simulink model "sampleModel7293_pp_1_1"  (R2018a)
settings: Solver=VariableStepAuto  StartTime=0.0  StopTime=10.0  RelTol=1e-3
undefined symbols (not defined in the file): DiscIntNeverNeededParam
libraries: simulink x367
(part 12 of 12)

== system sampleModel7293_pp_1_1/cfblk187/cfblk12/cfblk3 ==
  emi_1187 : Inport
  emi_1188 : Inport  Port=2
  Action Port : ActionPort  ActionType=then
  cfblk3 : simulink/Continuous/PID Controller (2DOF)  Controller=PID  TimeDomain=Discrete-time  SampleTime=-1  IntegratorMethod=Forward Euler  FilterMethod=Forward Euler  Form=Parallel  UseFilter=on  ControllerParametersSource=internal  P=1  I=1  D=0  N=100  b=1  c=1  InitialConditionSource=internal  InitialConditionForIntegrator=0  InitialConditionForFilter=0  ExternalReset=none  LimitOutput=off  UpperSaturationLimit=inf  LowerSaturationLimit=-inf  LinearizeAsGain=off  AntiWindupMode=none  Kb=1  TrackingMode=off  Kt=1  PParamMin=[]  PParamMax=[]  IParamMin=[]  IParamMax=[]  DParamMin=[]  DParamMax=[]  NParamMin=[]  NParamMax=[]  bParamMin=[]  bParamMax=[]  cParamMin=[]  cParamMax=[]  KbParamMin=[]  KbParamMax=[]  KtParamMin=[]  KtParamMax=[]  POutMin=[]  POutMax=[]  IOutMin=[]  IOutMax=[]  DOutMin=[]  DOutMax=[]  NOutMin=[]  NOutMax=[]  bOutMin=[]  bOutMax=[]  cOutMin=[]  cOutMax=[]  KbOutMin=[]  KbOutMax=[]  KtOutMin=[]  KtOutMax=[]  IntegratorOutMin=[]  IntegratorOutMax=[]  FilterOutMin=[]  FilterOutMax=[]  SumOutMin=[]  SumOutMax=[]  Sum1OutMin=[]  Sum1OutMax=[]  Sum2OutMin=[]  Sum2OutMax=[]  Sum3OutMin=[]  Sum3OutMax=[]  SumI1OutMin=[]  SumI1OutMax=[]  SumI2OutMin=[]  SumI2OutMax=[]  SumI3OutMin=[]  SumI3OutMax=[]  SumDOutMin=[]  SumDOutMax=[]  SaturationOutMin=[]  SaturationOutMax=[]  IntegratorContinuousStateAttributes=''  IntegratorStateMustResolveToSignalObject=off  IntegratorRTWStateStorageClass=Auto  FilterContinuousStateAttributes=''  FilterStateMustResolveToSignalObject=off  FilterRTWStateStorageClass=Auto  DifferentiatorICPrevScaledInput=0  DifferentiatorOutMin=[]  DifferentiatorOutMax=[]  FilterDiffOutCoefMin=[]  FilterDiffOutCoefMax=[]  SumDenOutMin=[]  SumDenOutMax=[]  SumNumOutMin=[]  SumNumOutMax=[]  ReciprocalOutMin=[]  ReciprocalOutMax=[]  DivideOutMin=[]  DivideOutMax=[]  TunerSelectOption=Transfer Function Based (PID Tuner App)
  emi_1189 : Outport
  wires:
  emi_1187/1 -> cfblk3/1
  emi_1188/1 -> cfblk3/2
  cfblk3/1 -> emi_1189/1

== system sampleModel7293_pp_1_1/cfblk187/cfblk12/cfblk7 ==
  emi_322 : Inport
  Action Port : ActionPort  ActionType=then
  cfblk7 : DiscreteTransferFcn
  emi_323 : Outport
  wires:
  emi_322/1 -> cfblk7/1
  cfblk7/1 -> emi_323/1

== system sampleModel7293_pp_1_1/cfblk187/cfblk12/emi_1190 ==
  Action Port : ActionPort  ActionType=else
  emi_1191 : Assertion

== system sampleModel7293_pp_1_1/cfblk187/cfblk12/emi_324 ==
  Action Port : ActionPort  ActionType=else
  emi_325 : Assertion

== system sampleModel7293_pp_1_1/cfblk189/cfblk16/cfblk8 ==
  emi_903 : Inport
  Action Port : ActionPort  ActionType=then
  cfblk8 : simulink/Discrete/Transfer Fcn First Order  PoleZ=0.95  ICPrevOutput=0.0  DoSatur=off
      settings: SourceProductName=Simulink
  emi_904 : Outport
  wires:
  emi_903/1 -> cfblk8/1
  cfblk8/1 -> emi_904/1

== system sampleModel7293_pp_1_1/cfblk189/cfblk16/emi_905 ==
  Action Port : ActionPort  ActionType=else
  emi_906 : Assertion

== system sampleModel7293_pp_1_1/cfblk189/cfblk17/cfblk13 ==
  emi_359 : Inport
  Action Port : ActionPort  ActionType=then
  cfblk13 : simulink/Discrete/Difference  ICPrevInput=0.0  OutMin=[]  OutMax=[]  OutDataTypeStr=double  OutputDataTypeScalingMode=double  OutDataType=fixdt(1, 16)  OutScaling=2^-10  DoSatur=off
  emi_360 : Outport
  wires:
  emi_359/1 -> cfblk13/1
  cfblk13/1 -> emi_360/1

== system sampleModel7293_pp_1_1/cfblk189/cfblk17/cfblk4 ==
  emi_810 : Inport
  Action Port : ActionPort  ActionType=then
  cfblk4 : DiscreteStateSpace  SampleTime=-1
  emi_811 : Outport
  wires:
  emi_810/1 -> cfblk4/1
  cfblk4/1 -> emi_811/1

== system sampleModel7293_pp_1_1/cfblk189/cfblk17/cfblk9 ==
  emi_366 : Inport
  Action Port : ActionPort  ActionType=then
  cfblk9 : DiscreteTransferFcn
  emi_367 : Outport
  wires:
  emi_366/1 -> cfblk9/1
  cfblk9/1 -> emi_367/1

== system sampleModel7293_pp_1_1/cfblk189/cfblk17/emi_361 ==
  Action Port : ActionPort  ActionType=else
  emi_362 : Assertion

== system sampleModel7293_pp_1_1/cfblk189/cfblk17/emi_368 ==
  Action Port : ActionPort  ActionType=else
  emi_369 : Assertion

== system sampleModel7293_pp_1_1/cfblk189/cfblk17/emi_812 ==
  Action Port : ActionPort  ActionType=else
  emi_813 : Assertion

== system sampleModel7293_pp_1_1/cfblk190/cfblk10/cfblk10 ==
  emi_523 : Inport
  emi_524 : Inport  Port=2
  Action Port : ActionPort  ActionType=then
  cfblk10 : Delay  DelayLengthSource=Input port
      settings: InputPortMap=u0,p1
  emi_525 : Outport
  wires:
  emi_523/1 -> cfblk10/1
  emi_524/1 -> cfblk10/2
  cfblk10/1 -> emi_525/1

== system sampleModel7293_pp_1_1/cfblk190/cfblk10/cfblk16 ==
  emi_545 : Inport
  Action Port : ActionPort  ActionType=then
  cfblk16 : Delay
  emi_546 : Outport
  wires:
  emi_545/1 -> cfblk16/1
  cfblk16/1 -> emi_546/1

== system sampleModel7293_pp_1_1/cfblk190/cfblk10/cfblk4 ==
  emi_952 : Inport
  Action Port : ActionPort  ActionType=then
  cfblk4 : DiscreteFir
  emi_953 : Outport
  wires:
  emi_952/1 -> cfblk4/1
  cfblk4/1 -> emi_953/1

== system sampleModel7293_pp_1_1/cfblk190/cfblk10/cfblk5 ==
  emi_1223 : Inport
  Action Port : ActionPort  ActionType=then
  cfblk5 : simulink/Continuous/PID Controller  Controller=PID  TimeDomain=Discrete-time  SampleTime=-1  IntegratorMethod=Forward Euler  FilterMethod=Forward Euler  Form=Parallel  UseFilter=on  ControllerParametersSource=internal  P=1  I=1  D=0  N=100  InitialConditionSource=internal  InitialConditionForIntegrator=0  InitialConditionForFilter=0  ExternalReset=none  LimitOutput=off  UpperSaturationLimit=inf  LowerSaturationLimit=-inf  LinearizeAsGain=off  AntiWindupMode=none  Kb=1  TrackingMode=off  Kt=1  PParamMin=[]  PParamMax=[]  IParamMin=[]  IParamMax=[]  DParamMin=[]  DParamMax=[]  NParamMin=[]  NParamMax=[]  KbParamMin=[]  KbParamMax=[]  KtParamMin=[]  KtParamMax=[]  POutMin=[]  POutMax=[]  IOutMin=[]  IOutMax=[]  DOutMin=[]  DOutMax=[]  NOutMin=[]  NOutMax=[]  KbOutMin=[]  KbOutMax=[]  KtOutMin=[]  KtOutMax=[]  IntegratorOutMin=[]  IntegratorOutMax=[]  FilterOutMin=[]  FilterOutMax=[]  SumOutMin=[]  SumOutMax=[]  SumI1OutMin=[]  SumI1OutMax=[]  SumI2OutMin=[]  SumI2OutMax=[]  SumI3OutMin=[]  SumI3OutMax=[]  SumDOutMin=[]  SumDOutMax=[]  SaturationOutMin=[]  SaturationOutMax=[]  IntegratorContinuousStateAttributes=''  IntegratorStateMustResolveToSignalObject=off  IntegratorRTWStateStorageClass=Auto  FilterContinuousStateAttributes=''  FilterStateMustResolveToSignalObject=off  FilterRTWStateStorageClass=Auto  DifferentiatorICPrevScaledInput=0  DifferentiatorOutMin=[]  DifferentiatorOutMax=[]  FilterDiffOutCoefMin=[]  FilterDiffOutCoefMax=[]  SumDenOutMin=[]  SumDenOutMax=[]  SumNumOutMin=[]  SumNumOutMax=[]  ReciprocalOutMin=[]  ReciprocalOutMax=[]  DivideOutMin=[]  DivideOutMax=[]  TunerSelectOption=Transfer Function Based (PID Tuner App)
  emi_1224 : Outport
  wires:
  emi_1223/1 -> cfblk5/1
  cfblk5/1 -> emi_1224/1

== system sampleModel7293_pp_1_1/cfblk190/cfblk10/cfblk8 ==
  emi_279 : Inport
  Action Port : ActionPort  ActionType=then
  cfblk8 : Delay
  emi_280 : Outport
  wires:
  emi_279/1 -> cfblk8/1
  cfblk8/1 -> emi_280/1

== system sampleModel7293_pp_1_1/cfblk190/cfblk10/cfblk9 ==
  emi_1871 : Inport
  Action Port : ActionPort  ActionType=then
  cfblk9 : DiscreteZeroPole  Poles=[0 0.5]  Gain=1  SampleTime=-1
  emi_1872 : Outport
  wires:
  emi_1871/1 -> cfblk9/1
  cfblk9/1 -> emi_1872/1

== system sampleModel7293_pp_1_1/cfblk190/cfblk10/emi_1225 ==
  Action Port : ActionPort  ActionType=else
  emi_1226 : Assertion

== system sampleModel7293_pp_1_1/cfblk190/cfblk10/emi_1873 ==
  Action Port : ActionPort  ActionType=else
  emi_1874 : Assertion

== system sampleModel7293_pp_1_1/cfblk190/cfblk10/emi_281 ==
  Action Port : ActionPort  ActionType=else
  emi_282 : Assertion

== system sampleModel7293_pp_1_1/cfblk190/cfblk10/emi_526 ==
  Action Port : ActionPort  ActionType=else
  emi_527 : Assertion

== system sampleModel7293_pp_1_1/cfblk190/cfblk10/emi_547 ==
  Action Port : ActionPort  ActionType=else
  emi_548 : Assertion

== system sampleModel7293_pp_1_1/cfblk190/cfblk10/emi_954 ==
  Action Port : ActionPort  ActionType=else
  emi_955 : Assertion

== system sampleModel7293_pp_1_1/cfblk190/cfblk9/cfblk10 ==
  emi_1057 : Inport
  Action Port : ActionPort  ActionType=then
  cfblk10 : DiscreteFilter
  emi_1058 : Outport
  wires:
  emi_1057/1 -> cfblk10/1
  cfblk10/1 -> emi_1058/1

== system sampleModel7293_pp_1_1/cfblk190/cfblk9/cfblk14 ==
  emi_1209 : Inport
  Action Port : ActionPort  ActionType=then
  cfblk14 : Delay
  emi_1210 : Outport
  wires:
  emi_1209/1 -> cfblk14/1
  cfblk14/1 -> emi_1210/1

== system sampleModel7293_pp_1_1/cfblk190/cfblk9/cfblk5 ==
  emi_1372 : Inport
  Action Port : ActionPort  ActionType=then
  cfblk5 : DiscreteZeroPole  Poles=[0 0.5]  Gain=1  SampleTime=-1
  emi_1373 : Outport
  wires:
  emi_1372/1 -> cfblk5/1
  cfblk5/1 -> emi_1373/1

== system sampleModel7293_pp_1_1/cfblk190/cfblk9/cfblk6 ==
  emi_688 : Inport
  Action Port : ActionPort  ActionType=then
  cfblk6 : DiscreteIntegrator  SampleTime=-1  OutDataTypeStr=double  ICPrevOutput=DiscIntNeverNeededParam  ICPrevScaledInput=DiscIntNeverNeededParam
  emi_689 : Outport
  wires:
  emi_688/1 -> cfblk6/1
  cfblk6/1 -> emi_689/1

== system sampleModel7293_pp_1_1/cfblk190/cfblk9/cfblk8 ==
  emi_1969 : Inport
  Action Port : ActionPort  ActionType=then
  cfblk8 : DiscreteFilter
  emi_1970 : Outport
  wires:
  emi_1969/1 -> cfblk8/1
  cfblk8/1 -> emi_1970/1

== system sampleModel7293_pp_1_1/cfblk190/cfblk9/emi_1059 ==
  Action Port : ActionPort  ActionType=else
  emi_1060 : Assertion

== system sampleModel7293_pp_1_1/cfblk190/cfblk9/emi_1211 ==
  Action Port : ActionPort  ActionType=else
  emi_1212 : Assertion

== system sampleModel7293_pp_1_1/cfblk190/cfblk9/emi_1374 ==
  Action Port : ActionPort  ActionType=else
  emi_1375 : Assertion

== system sampleModel7293_pp_1_1/cfblk190/cfblk9/emi_1971 ==
  Action Port : ActionPort  ActionType=else
  emi_1972 : Assertion

== system sampleModel7293_pp_1_1/cfblk190/cfblk9/emi_690 ==
  Action Port : ActionPort  ActionType=else
  emi_691 : Assertion

== system sampleModel7293_pp_1_1/cfblk193/cfblk17/cfblk6 ==
  emi_2054 : Inport
  Action Port : ActionPort  ActionType=then
  cfblk6 : DiscreteFilter
  emi_2055 : Outport
  wires:
  emi_2054/1 -> cfblk6/1
  cfblk6/1 -> emi_2055/1

== system sampleModel7293_pp_1_1/cfblk193/cfblk17/cfblk8 ==
  emi_22 : Inport
  Action Port : ActionPort  ActionType=then
  cfblk8 : simulink/Continuous/PID Controller  Controller=PID  TimeDomain=Discrete-time  SampleTime=-1  IntegratorMethod=Forward Euler  FilterMethod=Forward Euler  Form=Parallel  UseFilter=on  ControllerParametersSource=internal  P=1  I=1  D=0  N=100  InitialConditionSource=internal  InitialConditionForIntegrator=0  InitialConditionForFilter=0  ExternalReset=none  LimitOutput=off  UpperSaturationLimit=inf  LowerSaturationLimit=-inf  LinearizeAsGain=off  AntiWindupMode=none  Kb=1  TrackingMode=off  Kt=1  PParamMin=[]  PParamMax=[]  IParamMin=[]  IParamMax=[]  DParamMin=[]  DParamMax=[]  NParamMin=[]  NParamMax=[]  KbParamMin=[]  KbParamMax=[]  KtParamMin=[]  KtParamMax=[]  POutMin=[]  POutMax=[]  IOutMin=[]  IOutMax=[]  DOutMin=[]  DOutMax=[]  NOutMin=[]  NOutMax=[]  KbOutMin=[]  KbOutMax=[]  KtOutMin=[]  KtOutMax=[]  IntegratorOutMin=[]  IntegratorOutMax=[]  FilterOutMin=[]  FilterOutMax=[]  SumOutMin=[]  SumOutMax=[]  SumI1OutMin=[]  SumI1OutMax=[]  SumI2OutMin=[]  SumI2OutMax=[]  SumI3OutMin=[]  SumI3OutMax=[]  SumDOutMin=[]  SumDOutMax=[]  SaturationOutMin=[]  SaturationOutMax=[]  IntegratorContinuousStateAttributes=''  IntegratorStateMustResolveToSignalObject=off  IntegratorRTWStateStorageClass=Auto  FilterContinuousStateAttributes=''  FilterStateMustResolveToSignalObject=off  FilterRTWStateStorageClass=Auto  DifferentiatorICPrevScaledInput=0  DifferentiatorOutMin=[]  DifferentiatorOutMax=[]  FilterDiffOutCoefMin=[]  FilterDiffOutCoefMax=[]  SumDenOutMin=[]  SumDenOutMax=[]  SumNumOutMin=[]  SumNumOutMax=[]  ReciprocalOutMin=[]  ReciprocalOutMax=[]  DivideOutMin=[]  DivideOutMax=[]  TunerSelectOption=Transfer Function Based (PID Tuner App)
  emi_23 : Outport
  wires:
  emi_22/1 -> cfblk8/1
  cfblk8/1 -> emi_23/1

== system sampleModel7293_pp_1_1/cfblk193/cfblk17/emi_2056 ==
  Action Port : ActionPort  ActionType=else
  emi_2057 : Assertion

== system sampleModel7293_pp_1_1/cfblk193/cfblk17/emi_24 ==
  Action Port : ActionPort  ActionType=else
  emi_25 : Assertion

== system sampleModel7293_pp_1_1/cfblk193/cfblk19/cfblk18 ==
  emi_695 : Inport
  Action Port : ActionPort  ActionType=then
  cfblk18 : Delay
  emi_696 : Outport
  wires:
  emi_695/1 -> cfblk18/1
  cfblk18/1 -> emi_696/1

== system sampleModel7293_pp_1_1/cfblk193/cfblk19/emi_697 ==
  Action Port : ActionPort  ActionType=else
  emi_698 : Assertion

== system sampleModel7293_pp_1_1/cfblk193/cfblk20/cfblk10 ==
  emi_538 : Inport
  Action Port : ActionPort  ActionType=then
  cfblk10 : DiscreteFilter
  emi_539 : Outport
  wires:
  emi_538/1 -> cfblk10/1
  cfblk10/1 -> emi_539/1

== system sampleModel7293_pp_1_1/cfblk193/cfblk20/cfblk4 ==
  emi_222 : Inport
  Action Port : ActionPort  ActionType=then
  cfblk4 : simulink/Discrete/Transfer Fcn First Order  PoleZ=0.95  ICPrevOutput=0.0  DoSatur=off
      settings: SourceProductName=Simulink
  emi_223 : Outport
  wires:
  emi_222/1 -> cfblk4/1
  cfblk4/1 -> emi_223/1

== system sampleModel7293_pp_1_1/cfblk193/cfblk20/cfblk7 ==
  emi_610 : Inport
  Action Port : ActionPort  ActionType=then
  cfblk7 : DiscreteFilter
  emi_611 : Outport
  wires:
  emi_610/1 -> cfblk7/1
  cfblk7/1 -> emi_611/1

== system sampleModel7293_pp_1_1/cfblk193/cfblk20/emi_224 ==
  Action Port : ActionPort  ActionType=else
  emi_225 : Assertion

== system sampleModel7293_pp_1_1/cfblk193/cfblk20/emi_540 ==
  Action Port : ActionPort  ActionType=else
  emi_541 : Assertion

== system sampleModel7293_pp_1_1/cfblk193/cfblk20/emi_612 ==
  Action Port : ActionPort  ActionType=else
  emi_613 : Assertion

== system sampleModel7293_pp_1_1/cfblk195/cfblk8/cfblk13 ==
  emi_1593 : Inport
  Action Port : ActionPort  ActionType=then
  cfblk13 : Delay
  emi_1594 : Outport
  wires:
  emi_1593/1 -> cfblk13/1
  cfblk13/1 -> emi_1594/1

== system sampleModel7293_pp_1_1/cfblk195/cfblk8/cfblk8 ==
  emi_495 : Inport
  Action Port : ActionPort  ActionType=then
  cfblk8 : DiscreteZeroPole  Poles=[0 0.5]  Gain=1  SampleTime=-1
  emi_496 : Outport
  wires:
  emi_495/1 -> cfblk8/1
  cfblk8/1 -> emi_496/1

== system sampleModel7293_pp_1_1/cfblk195/cfblk8/cfblk9 ==
  emi_1991 : Inport
  Action Port : ActionPort  ActionType=then
  cfblk9 : DiscreteStateSpace  SampleTime=-1
  emi_1992 : Outport
  wires:
  emi_1991/1 -> cfblk9/1
  cfblk9/1 -> emi_1992/1

== system sampleModel7293_pp_1_1/cfblk195/cfblk8/emi_1595 ==
  Action Port : ActionPort  ActionType=else
  emi_1596 : Assertion

== system sampleModel7293_pp_1_1/cfblk195/cfblk8/emi_1993 ==
  Action Port : ActionPort  ActionType=else
  emi_1994 : Assertion

== system sampleModel7293_pp_1_1/cfblk195/cfblk8/emi_497 ==
  Action Port : ActionPort  ActionType=else
  emi_498 : Assertion

== system sampleModel7293_pp_1_1/cfblk195/cfblk9/cfblk9 ==
  emi_1586 : Inport
  Action Port : ActionPort  ActionType=then
  cfblk9 : simulink/Continuous/PID Controller  Controller=PID  TimeDomain=Discrete-time  SampleTime=-1  IntegratorMethod=Forward Euler  FilterMethod=Forward Euler  Form=Parallel  UseFilter=on  ControllerParametersSource=internal  P=1  I=1  D=0  N=100  InitialConditionSource=internal  InitialConditionForIntegrator=0  InitialConditionForFilter=0  ExternalReset=none  LimitOutput=off  UpperSaturationLimit=inf  LowerSaturationLimit=-inf  LinearizeAsGain=off  AntiWindupMode=none  Kb=1  TrackingMode=off  Kt=1  PParamMin=[]  PParamMax=[]  IParamMin=[]  IParamMax=[]  DParamMin=[]  DParamMax=[]  NParamMin=[]  NParamMax=[]  KbParamMin=[]  KbParamMax=[]  KtParamMin=[]  KtParamMax=[]  POutMin=[]  POutMax=[]  IOutMin=[]  IOutMax=[]  DOutMin=[]  DOutMax=[]  NOutMin=[]  NOutMax=[]  KbOutMin=[]  KbOutMax=[]  KtOutMin=[]  KtOutMax=[]  IntegratorOutMin=[]  IntegratorOutMax=[]  FilterOutMin=[]  FilterOutMax=[]  SumOutMin=[]  SumOutMax=[]  SumI1OutMin=[]  SumI1OutMax=[]  SumI2OutMin=[]  SumI2OutMax=[]  SumI3OutMin=[]  SumI3OutMax=[]  SumDOutMin=[]  SumDOutMax=[]  SaturationOutMin=[]  SaturationOutMax=[]  IntegratorContinuousStateAttributes=''  IntegratorStateMustResolveToSignalObject=off  IntegratorRTWStateStorageClass=Auto  FilterContinuousStateAttributes=''  FilterStateMustResolveToSignalObject=off  FilterRTWStateStorageClass=Auto  DifferentiatorICPrevScaledInput=0  DifferentiatorOutMin=[]  DifferentiatorOutMax=[]  FilterDiffOutCoefMin=[]  FilterDiffOutCoefMax=[]  SumDenOutMin=[]  SumDenOutMax=[]  SumNumOutMin=[]  SumNumOutMax=[]  ReciprocalOutMin=[]  ReciprocalOutMax=[]  DivideOutMin=[]  DivideOutMax=[]  TunerSelectOption=Transfer Function Based (PID Tuner App)
  emi_1587 : Outport
  wires:
  emi_1586/1 -> cfblk9/1
  cfblk9/1 -> emi_1587/1

== system sampleModel7293_pp_1_1/cfblk195/cfblk9/emi_1588 ==
  Action Port : ActionPort  ActionType=else
  emi_1589 : Assertion

== system sampleModel7293_pp_1_1/cfblk196/cfblk11/cfblk3 ==
  emi_1150 : Inport
  Action Port : ActionPort  ActionType=then
  cfblk3 : DiscreteStateSpace  SampleTime=-1
  emi_1151 : Outport
  wires:
  emi_1150/1 -> cfblk3/1
  cfblk3/1 -> emi_1151/1

== system sampleModel7293_pp_1_1/cfblk196/cfblk11/emi_1152 ==
  Action Port : ActionPort  ActionType=else
  emi_1153 : Assertion

== system sampleModel7293_pp_1_1/cfblk196/cfblk12/cfblk3 ==
  emi_1821 : Inport
  Action Port : ActionPort  ActionType=then
  cfblk3 : simulink/Continuous/PID Controller  Controller=PID  TimeDomain=Discrete-time  SampleTime=-1  IntegratorMethod=Forward Euler  FilterMethod=Forward Euler  Form=Parallel  UseFilter=on  ControllerParametersSource=internal  P=1  I=1  D=0  N=100  InitialConditionSource=internal  InitialConditionForIntegrator=0  InitialConditionForFilter=0  ExternalReset=none  LimitOutput=off  UpperSaturationLimit=inf  LowerSaturationLimit=-inf  LinearizeAsGain=off  AntiWindupMode=none  Kb=1  TrackingMode=off  Kt=1  PParamMin=[]  PParamMax=[]  IParamMin=[]  IParamMax=[]  DParamMin=[]  DParamMax=[]  NParamMin=[]  NParamMax=[]  KbParamMin=[]  KbParamMax=[]  KtParamMin=[]  KtParamMax=[]  POutMin=[]  POutMax=[]  IOutMin=[]  IOutMax=[]  DOutMin=[]  DOutMax=[]  NOutMin=[]  NOutMax=[]  KbOutMin=[]  KbOutMax=[]  KtOutMin=[]  KtOutMax=[]  IntegratorOutMin=[]  IntegratorOutMax=[]  FilterOutMin=[]  FilterOutMax=[]  SumOutMin=[]  SumOutMax=[]  SumI1OutMin=[]  SumI1OutMax=[]  SumI2OutMin=[]  SumI2OutMax=[]  SumI3OutMin=[]  SumI3OutMax=[]  SumDOutMin=[]  SumDOutMax=[]  SaturationOutMin=[]  SaturationOutMax=[]  IntegratorContinuousStateAttributes=''  IntegratorStateMustResolveToSignalObject=off  IntegratorRTWStateStorageClass=Auto  FilterContinuousStateAttributes=''  FilterStateMustResolveToSignalObject=off  FilterRTWStateStorageClass=Auto  DifferentiatorICPrevScaledInput=0  DifferentiatorOutMin=[]  DifferentiatorOutMax=[]  FilterDiffOutCoefMin=[]  FilterDiffOutCoefMax=[]  SumDenOutMin=[]  SumDenOutMax=[]  SumNumOutMin=[]  SumNumOutMax=[]  ReciprocalOutMin=[]  ReciprocalOutMax=[]  DivideOutMin=[]  DivideOutMax=[]  TunerSelectOption=Transfer Function Based (PID Tuner App)
  emi_1822 : Outport
  wires:
  emi_1821/1 -> cfblk3/1
  cfblk3/1 -> emi_1822/1

== system sampleModel7293_pp_1_1/cfblk196/cfblk12/cfblk9 ==
  emi_567 : Inport
  Action Port : ActionPort  ActionType=then
  cfblk9 : DiscreteStateSpace  SampleTime=-1
  emi_568 : Outport
  wires:
  emi_567/1 -> cfblk9/1
  cfblk9/1 -> emi_568/1

== system sampleModel7293_pp_1_1/cfblk196/cfblk12/emi_1823 ==
  Action Port : ActionPort  ActionType=else
  emi_1824 : Assertion

== system sampleModel7293_pp_1_1/cfblk196/cfblk12/emi_569 ==
  Action Port : ActionPort  ActionType=else
  emi_570 : Assertion

== system sampleModel7293_pp_1_1/cfblk197/cfblk16/cfblk4 ==
  emi_1885 : Inport
  Action Port : ActionPort  ActionType=then
  cfblk4 : DiscreteTransferFcn
  emi_1886 : Outport
  wires:
  emi_1885/1 -> cfblk4/1
  cfblk4/1 -> emi_1886/1

== system sampleModel7293_pp_1_1/cfblk197/cfblk16/cfblk9 ==
  emi_1450 : Inport
  Action Port : ActionPort  ActionType=then
  cfblk9 : UnitDelay  SampleTime=-1
  emi_1451 : Outport
  wires:
  emi_1450/1 -> cfblk9/1
  cfblk9/1 -> emi_1451/1

== system sampleModel7293_pp_1_1/cfblk197/cfblk16/emi_1452 ==
  Action Port : ActionPort  ActionType=else
  emi_1453 : Assertion

== system sampleModel7293_pp_1_1/cfblk197/cfblk16/emi_1887 ==
  Action Port : ActionPort  ActionType=else
  emi_1888 : Assertion

== system sampleModel7293_pp_1_1/cfblk197/cfblk17/cfblk16 ==
  emi_1779 : Inport
  Action Port : ActionPort  ActionType=then
  cfblk16 : Delay
  emi_1780 : Outport
  wires:
  emi_1779/1 -> cfblk16/1
  cfblk16/1 -> emi_1780/1

== system sampleModel7293_pp_1_1/cfblk197/cfblk17/cfblk4 ==
  emi_1323 : Inport
  Action Port : ActionPort  ActionType=then
  cfblk4 : DiscreteZeroPole  Poles=[0 0.5]  Gain=1  SampleTime=-1
  emi_1324 : Outport
  wires:
  emi_1323/1 -> cfblk4/1
  cfblk4/1 -> emi_1324/1

== system sampleModel7293_pp_1_1/cfblk197/cfblk17/cfblk6 ==
  emi_767 : Inport
  Action Port : ActionPort  ActionType=then
  cfblk6 : simulink/Discrete/Difference  ICPrevInput=0.0  OutMin=[]  OutMax=[]  OutDataTypeStr=double  OutputDataTypeScalingMode=double  OutDataType=fixdt(1, 16)  OutScaling=2^-10  DoSatur=off
  emi_768 : Outport
  wires:
  emi_767/1 -> cfblk6/1
  cfblk6/1 -> emi_768/1

== system sampleModel7293_pp_1_1/cfblk197/cfblk17/emi_1325 ==
  Action Port : ActionPort  ActionType=else
  emi_1326 : Assertion

== system sampleModel7293_pp_1_1/cfblk197/cfblk17/emi_1781 ==
  Action Port : ActionPort  ActionType=else
  emi_1782 : Assertion

== system sampleModel7293_pp_1_1/cfblk197/cfblk17/emi_769 ==
  Action Port : ActionPort  ActionType=else
  emi_770 : Assertion

== system sampleModel7293_pp_1_1/cfblk198/cfblk14/cfblk7 ==
  emi_1429 : Inport
  Action Port : ActionPort  ActionType=then
  cfblk7 : DiscreteFir
  emi_1430 : Outport
  wires:
  emi_1429/1 -> cfblk7/1
  cfblk7/1 -> emi_1430/1

== system sampleModel7293_pp_1_1/cfblk198/cfblk14/cfblk9 ==
  emi_1707 : Inport
  Action Port : ActionPort  ActionType=then
  cfblk9 : simulink/Discrete/Tapped Delay  vinit=0.0  samptime=-1  NumDelays=1  DelayOrder=Oldest  includeCurrent=off
  emi_1708 : Outport
  wires:
  emi_1707/1 -> cfblk9/1
  cfblk9/1 -> emi_1708/1

== system sampleModel7293_pp_1_1/cfblk198/cfblk14/emi_1431 ==
  Action Port : ActionPort  ActionType=else
  emi_1432 : Assertion

== system sampleModel7293_pp_1_1/cfblk198/cfblk14/emi_1709 ==
  Action Port : ActionPort  ActionType=else
  emi_1710 : Assertion

== system sampleModel7293_pp_1_1/cfblk198/cfblk15/cfblk5 ==
  emi_2126 : Inport
  Action Port : ActionPort  ActionType=then
  cfblk5 : simulink/Discrete/Transfer Fcn First Order  PoleZ=0.95  ICPrevOutput=0.0  DoSatur=off
      settings: SourceProductName=Simulink
  emi_2127 : Outport
  wires:
  emi_2126/1 -> cfblk5/1
  cfblk5/1 -> emi_2127/1

== system sampleModel7293_pp_1_1/cfblk198/cfblk15/emi_2128 ==
  Action Port : ActionPort  ActionType=else
  emi_2129 : Assertion

== system sampleModel7293_pp_1_1/cfblk198/cfblk16/cfblk11 ==
  emi_1892 : Inport
  Action Port : ActionPort  ActionType=then
  cfblk11 : simulink/Discrete/Tapped Delay  vinit=0.0  samptime=-1  NumDelays=1  DelayOrder=Oldest  includeCurrent=off
  emi_1893 : Outport
  wires:
  emi_1892/1 -> cfblk11/1
  cfblk11/1 -> emi_1893/1

== system sampleModel7293_pp_1_1/cfblk198/cfblk16/cfblk13 ==
  emi_164 : Inport
  Action Port : ActionPort  ActionType=then
  cfblk13 : DiscreteFilter
  emi_165 : Outport
  wires:
  emi_164/1 -> cfblk13/1
  cfblk13/1 -> emi_165/1

== system sampleModel7293_pp_1_1/cfblk198/cfblk16/cfblk16 ==
  emi_725 : Inport
  Action Port : ActionPort  ActionType=then
  cfblk16 : Delay
  emi_726 : Outport
  wires:
  emi_725/1 -> cfblk16/1
  cfblk16/1 -> emi_726/1

== system sampleModel7293_pp_1_1/cfblk198/cfblk16/cfblk17 ==
  emi_1015 : Inport
  Action Port : ActionPort  ActionType=then
  cfblk17 : Delay
  emi_1016 : Outport
  wires:
  emi_1015/1 -> cfblk17/1
  cfblk17/1 -> emi_1016/1

== system sampleModel7293_pp_1_1/cfblk198/cfblk16/cfblk4 ==
  emi_1315 : Inport
  emi_1316 : Inport  Port=2
  Action Port : ActionPort  ActionType=then
  cfblk4 : Delay  DelayLengthSource=Input port
      settings: InputPortMap=u0,p1
  emi_1317 : Outport
  wires:
  emi_1315/1 -> cfblk4/1
  emi_1316/1 -> cfblk4/2
  cfblk4/1 -> emi_1317/1

== system sampleModel7293_pp_1_1/cfblk198/cfblk16/emi_1017 ==
  Action Port : ActionPort  ActionType=else
  emi_1018 : Assertion

== system sampleModel7293_pp_1_1/cfblk198/cfblk16/emi_1318 ==
  Action Port : ActionPort  ActionType=else
  emi_1319 : Assertion

== system sampleModel7293_pp_1_1/cfblk198/cfblk16/emi_166 ==
  Action Port : ActionPort  ActionType=else
  emi_167 : Assertion

== system sampleModel7293_pp_1_1/cfblk198/cfblk16/emi_1894 ==
  Action Port : ActionPort  ActionType=else
  emi_1895 : Assertion

== system sampleModel7293_pp_1_1/cfblk198/cfblk16/emi_727 ==
  Action Port : ActionPort  ActionType=else
  emi_728 : Assertion

== system sampleModel7293_pp_1_1/cfblk198/cfblk17/cfblk6 ==
  emi_1607 : Inport
  Action Port : ActionPort  ActionType=then
  cfblk6 : DiscreteZeroPole  Poles=[0 0.5]  Gain=1  SampleTime=-1
  emi_1608 : Outport
  wires:
  emi_1607/1 -> cfblk6/1
  cfblk6/1 -> emi_1608/1

== system sampleModel7293_pp_1_1/cfblk198/cfblk17/cfblk9 ==
  emi_443 : Inport
  Action Port : ActionPort  ActionType=then
  cfblk9 : DiscreteStateSpace  SampleTime=-1
  emi_444 : Outport
  wires:
  emi_443/1 -> cfblk9/1
  cfblk9/1 -> emi_444/1

== system sampleModel7293_pp_1_1/cfblk198/cfblk17/emi_1609 ==
  Action Port : ActionPort  ActionType=else
  emi_1610 : Assertion

== system sampleModel7293_pp_1_1/cfblk198/cfblk17/emi_445 ==
  Action Port : ActionPort  ActionType=else
  emi_446 : Assertion

== system sampleModel7293_pp_1_1/cfblk198/cfblk18/cfblk12 ==
  emi_1457 : Inport
  Action Port : ActionPort  ActionType=then
  cfblk12 : simulink/Continuous/PID Controller  Controller=PID  TimeDomain=Discrete-time  SampleTime=-1  IntegratorMethod=Forward Euler  FilterMethod=Forward Euler  Form=Parallel  UseFilter=on  ControllerParametersSource=internal  P=1  I=1  D=0  N=100  InitialConditionSource=internal  InitialConditionForIntegrator=0  InitialConditionForFilter=0  ExternalReset=none  LimitOutput=off  UpperSaturationLimit=inf  LowerSaturationLimit=-inf  LinearizeAsGain=off  AntiWindupMode=none  Kb=1  TrackingMode=off  Kt=1  PParamMin=[]  PParamMax=[]  IParamMin=[]  IParamMax=[]  DParamMin=[]  DParamMax=[]  NParamMin=[]  NParamMax=[]  KbParamMin=[]  KbParamMax=[]  KtParamMin=[]  KtParamMax=[]  POutMin=[]  POutMax=[]  IOutMin=[]  IOutMax=[]  DOutMin=[]  DOutMax=[]  NOutMin=[]  NOutMax=[]  KbOutMin=[]  KbOutMax=[]  KtOutMin=[]  KtOutMax=[]  IntegratorOutMin=[]  IntegratorOutMax=[]  FilterOutMin=[]  FilterOutMax=[]  SumOutMin=[]  SumOutMax=[]  SumI1OutMin=[]  SumI1OutMax=[]  SumI2OutMin=[]  SumI2OutMax=[]  SumI3OutMin=[]  SumI3OutMax=[]  SumDOutMin=[]  SumDOutMax=[]  SaturationOutMin=[]  SaturationOutMax=[]  IntegratorContinuousStateAttributes=''  IntegratorStateMustResolveToSignalObject=off  IntegratorRTWStateStorageClass=Auto  FilterContinuousStateAttributes=''  FilterStateMustResolveToSignalObject=off  FilterRTWStateStorageClass=Auto  DifferentiatorICPrevScaledInput=0  DifferentiatorOutMin=[]  DifferentiatorOutMax=[]  FilterDiffOutCoefMin=[]  FilterDiffOutCoefMax=[]  SumDenOutMin=[]  SumDenOutMax=[]  SumNumOutMin=[]  SumNumOutMax=[]  ReciprocalOutMin=[]  ReciprocalOutMax=[]  DivideOutMin=[]  DivideOutMax=[]  TunerSelectOption=Transfer Function Based (PID Tuner App)
  emi_1458 : Outport
  wires:
  emi_1457/1 -> cfblk12/1
  cfblk12/1 -> emi_1458/1

== system sampleModel7293_pp_1_1/cfblk198/cfblk18/cfblk13 ==
  emi_1344 : Inport
  Action Port : ActionPort  ActionType=then
  cfblk13 : DiscreteZeroPole  Poles=[0 0.5]  Gain=1  SampleTime=-1
  emi_1345 : Outport
  wires:
  emi_1344/1 -> cfblk13/1
  cfblk13/1 -> emi_1345/1

== system sampleModel7293_pp_1_1/cfblk198/cfblk18/cfblk5 ==
  emi_574 : Inport
  Action Port : ActionPort  ActionType=then
  cfblk5 : UnitDelay  SampleTime=-1
  emi_575 : Outport
  wires:
  emi_574/1 -> cfblk5/1
  cfblk5/1 -> emi_575/1

== system sampleModel7293_pp_1_1/cfblk198/cfblk18/cfblk9 ==
  emi_1643 : Inport
  Action Port : ActionPort  ActionType=then
  cfblk9 : DiscreteIntegrator  SampleTime=-1  OutDataTypeStr=double  ICPrevOutput=DiscIntNeverNeededParam  ICPrevScaledInput=DiscIntNeverNeededParam
  emi_1644 : Outport
  wires:
  emi_1643/1 -> cfblk9/1
  cfblk9/1 -> emi_1644/1

== system sampleModel7293_pp_1_1/cfblk198/cfblk18/emi_1346 ==
  Action Port : ActionPort  ActionType=else
  emi_1347 : Assertion

== system sampleModel7293_pp_1_1/cfblk198/cfblk18/emi_1459 ==
  Action Port : ActionPort  ActionType=else
  emi_1460 : Assertion

== system sampleModel7293_pp_1_1/cfblk198/cfblk18/emi_1645 ==
  Action Port : ActionPort  ActionType=else
  emi_1646 : Assertion

== system sampleModel7293_pp_1_1/cfblk198/cfblk18/emi_576 ==
  Action Port : ActionPort  ActionType=else
  emi_577 : Assertion

== system sampleModel7293_pp_1_1/cfblk198/cfblk19/cfblk7 ==
  emi_875 : Inport
  Action Port : ActionPort  ActionType=then
  cfblk7 : simulink/Continuous/PID Controller  Controller=PID  TimeDomain=Discrete-time  SampleTime=-1  IntegratorMethod=Forward Euler  FilterMethod=Forward Euler  Form=Parallel  UseFilter=on  ControllerParametersSource=internal  P=1  I=1  D=0  N=100  InitialConditionSource=internal  InitialConditionForIntegrator=0  InitialConditionForFilter=0  ExternalReset=none  LimitOutput=off  UpperSaturationLimit=inf  LowerSaturationLimit=-inf  LinearizeAsGain=off  AntiWindupMode=none  Kb=1  TrackingMode=off  Kt=1  PParamMin=[]  PParamMax=[]  IParamMin=[]  IParamMax=[]  DParamMin=[]  DParamMax=[]  NParamMin=[]  NParamMax=[]  KbParamMin=[]  KbParamMax=[]  KtParamMin=[]  KtParamMax=[]  POutMin=[]  POutMax=[]  IOutMin=[]  IOutMax=[]  DOutMin=[]  DOutMax=[]  NOutMin=[]  NOutMax=[]  KbOutMin=[]  KbOutMax=[]  KtOutMin=[]  KtOutMax=[]  IntegratorOutMin=[]  IntegratorOutMax=[]  FilterOutMin=[]  FilterOutMax=[]  SumOutMin=[]  SumOutMax=[]  SumI1OutMin=[]  SumI1OutMax=[]  SumI2OutMin=[]  SumI2OutMax=[]  SumI3OutMin=[]  SumI3OutMax=[]  SumDOutMin=[]  SumDOutMax=[]  SaturationOutMin=[]  SaturationOutMax=[]  IntegratorContinuousStateAttributes=''  IntegratorStateMustResolveToSignalObject=off  IntegratorRTWStateStorageClass=Auto  FilterContinuousStateAttributes=''  FilterStateMustResolveToSignalObject=off  FilterRTWStateStorageClass=Auto  DifferentiatorICPrevScaledInput=0  DifferentiatorOutMin=[]  DifferentiatorOutMax=[]  FilterDiffOutCoefMin=[]  FilterDiffOutCoefMax=[]  SumDenOutMin=[]  SumDenOutMax=[]  SumNumOutMin=[]  SumNumOutMax=[]  ReciprocalOutMin=[]  ReciprocalOutMax=[]  DivideOutMin=[]  DivideOutMax=[]  TunerSelectOption=Transfer Function Based (PID Tuner App)
  emi_876 : Outport
  wires:
  emi_875/1 -> cfblk7/1
  cfblk7/1 -> emi_876/1

== system sampleModel7293_pp_1_1/cfblk198/cfblk19/emi_877 ==
  Action Port : ActionPort  ActionType=else
  emi_878 : Assertion

== system sampleModel7293_pp_1_1/cfblk199/cfblk12/cfblk5 ==
  emi_732 : Inport
  Action Port : ActionPort  ActionType=then
  cfblk5 : DiscreteTransferFcn
  emi_733 : Outport
  wires:
  emi_732/1 -> cfblk5/1
  cfblk5/1 -> emi_733/1

== system sampleModel7293_pp_1_1/cfblk199/cfblk12/cfblk7 ==
  emi_1679 : Inport
  Action Port : ActionPort  ActionType=then
  cfblk7 : simulink/Discrete/Transfer Fcn Lead or Lag  PoleZ=0.95  ZeroZ=0.75  ICPrevOutput=0.0  ICPrevInput=0.0  DoSatur=off
      settings: SourceProductName=Simulink  SourceProductBaseCode=SL
  emi_1680 : Outport
  wires:
  emi_1679/1 -> cfblk7/1
  cfblk7/1 -> emi_1680/1

== system sampleModel7293_pp_1_1/cfblk199/cfblk12/emi_1681 ==
  Action Port : ActionPort  ActionType=else
  emi_1682 : Assertion

== system sampleModel7293_pp_1_1/cfblk199/cfblk12/emi_734 ==
  Action Port : ActionPort  ActionType=else
  emi_735 : Assertion

== system sampleModel7293_pp_1_1/cfblk200/cfblk11/cfblk3 ==
  emi_966 : Inport
  Action Port : ActionPort  ActionType=then
  cfblk3 : DiscreteIntegrator  SampleTime=-1  OutDataTypeStr=double  ICPrevOutput=DiscIntNeverNeededParam  ICPrevScaledInput=DiscIntNeverNeededParam
  emi_967 : Outport
  wires:
  emi_966/1 -> cfblk3/1
  cfblk3/1 -> emi_967/1

== system sampleModel7293_pp_1_1/cfblk200/cfblk11/cfblk7 ==
  emi_994 : Inport
  Action Port : ActionPort  ActionType=then
  cfblk7 : simulink/Discrete/Tapped Delay  vinit=0.0  samptime=-1  NumDelays=1  DelayOrder=Oldest  includeCurrent=off
  emi_995 : Outport
  wires:
  emi_994/1 -> cfblk7/1
  cfblk7/1 -> emi_995/1

== system sampleModel7293_pp_1_1/cfblk200/cfblk11/emi_968 ==
  Action Port : ActionPort  ActionType=else
  emi_969 : Assertion

== system sampleModel7293_pp_1_1/cfblk200/cfblk11/emi_996 ==
  Action Port : ActionPort  ActionType=else
  emi_997 : Assertion

== system sampleModel7293_pp_1_1/cfblk200/cfblk12/cfblk10 ==
  emi_1273 : Inport
  Action Port : ActionPort  ActionType=then
  cfblk10 : Delay
  emi_1274 : Outport
  wires:
  emi_1273/1 -> cfblk10/1
  cfblk10/1 -> emi_1274/1

== system sampleModel7293_pp_1_1/cfblk200/cfblk12/cfblk11 ==
  emi_1114 : Inport
  Action Port : ActionPort  ActionType=then
  cfblk11 : Delay
  emi_1115 : Outport
  wires:
  emi_1114/1 -> cfblk11/1
  cfblk11/1 -> emi_1115/1

== system sampleModel7293_pp_1_1/cfblk200/cfblk12/cfblk3 ==
  emi_861 : Inport
  Action Port : ActionPort  ActionType=then
  cfblk3 : DiscreteZeroPole  Poles=[0 0.5]  Gain=1  SampleTime=-1
  emi_862 : Outport
  wires:
  emi_861/1 -> cfblk3/1
  cfblk3/1 -> emi_862/1

== system sampleModel7293_pp_1_1/cfblk200/cfblk12/cfblk4 ==
  emi_286 : Inport
  emi_287 : Inport  Port=2
  Action Port : ActionPort  ActionType=then
  cfblk4 : simulink/Continuous/PID Controller (2DOF)  Controller=PID  TimeDomain=Discrete-time  SampleTime=-1  IntegratorMethod=Forward Euler  FilterMethod=Forward Euler  Form=Parallel  UseFilter=on  ControllerParametersSource=internal  P=1  I=1  D=0  N=100  b=1  c=1  InitialConditionSource=internal  InitialConditionForIntegrator=0  InitialConditionForFilter=0  ExternalReset=none  LimitOutput=off  UpperSaturationLimit=inf  LowerSaturationLimit=-inf  LinearizeAsGain=off  AntiWindupMode=none  Kb=1  TrackingMode=off  Kt=1  PParamMin=[]  PParamMax=[]  IParamMin=[]  IParamMax=[]  DParamMin=[]  DParamMax=[]  NParamMin=[]  NParamMax=[]  bParamMin=[]  bParamMax=[]  cParamMin=[]  cParamMax=[]  KbParamMin=[]  KbParamMax=[]  KtParamMin=[]  KtParamMax=[]  POutMin=[]  POutMax=[]  IOutMin=[]  IOutMax=[]  DOutMin=[]  DOutMax=[]  NOutMin=[]  NOutMax=[]  bOutMin=[]  bOutMax=[]  cOutMin=[]  cOutMax=[]  KbOutMin=[]  KbOutMax=[]  KtOutMin=[]  KtOutMax=[]  IntegratorOutMin=[]  IntegratorOutMax=[]  FilterOutMin=[]  FilterOutMax=[]  SumOutMin=[]  SumOutMax=[]  Sum1OutMin=[]  Sum1OutMax=[]  Sum2OutMin=[]  Sum2OutMax=[]  Sum3OutMin=[]  Sum3OutMax=[]  SumI1OutMin=[]  SumI1OutMax=[]  SumI2OutMin=[]  SumI2OutMax=[]  SumI3OutMin=[]  SumI3OutMax=[]  SumDOutMin=[]  SumDOutMax=[]  SaturationOutMin=[]  SaturationOutMax=[]  IntegratorContinuousStateAttributes=''  IntegratorStateMustResolveToSignalObject=off  IntegratorRTWStateStorageClass=Auto  FilterContinuousStateAttributes=''  FilterStateMustResolveToSignalObject=off  FilterRTWStateStorageClass=Auto  DifferentiatorICPrevScaledInput=0  DifferentiatorOutMin=[]  DifferentiatorOutMax=[]  FilterDiffOutCoefMin=[]  FilterDiffOutCoefMax=[]  SumDenOutMin=[]  SumDenOutMax=[]  SumNumOutMin=[]  SumNumOutMax=[]  ReciprocalOutMin=[]  ReciprocalOutMax=[]  DivideOutMin=[]  DivideOutMax=[]  TunerSelectOption=Transfer Function Based (PID Tuner App)
  emi_288 : Outport
  wires:
  emi_286/1 -> cfblk4/1
  emi_287/1 -> cfblk4/2
  cfblk4/1 -> emi_288/1

== system sampleModel7293_pp_1_1/cfblk200/cfblk12/emi_1116 ==
  Action Port : ActionPort  ActionType=else
  emi_1117 : Assertion

== system sampleModel7293_pp_1_1/cfblk200/cfblk12/emi_1275 ==
  Action Port : ActionPort  ActionType=else
  emi_1276 : Assertion

== system sampleModel7293_pp_1_1/cfblk200/cfblk12/emi_289 ==
  Action Port : ActionPort  ActionType=else
  emi_290 : Assertion

== system sampleModel7293_pp_1_1/cfblk200/cfblk12/emi_863 ==
  Action Port : ActionPort  ActionType=else
  emi_864 : Assertion

== system sampleModel7293_pp_1_1/cfblk203/cfblk12/cfblk10 ==
  emi_1266 : Inport
  Action Port : ActionPort  ActionType=then
  cfblk10 : Delay
  emi_1267 : Outport
  wires:
  emi_1266/1 -> cfblk10/1
  cfblk10/1 -> emi_1267/1

== system sampleModel7293_pp_1_1/cfblk203/cfblk12/cfblk3 ==
  emi_788 : Inport
  Action Port : ActionPort  ActionType=then
  cfblk3 : DiscreteStateSpace  SampleTime=-1
  emi_789 : Outport
  wires:
  emi_788/1 -> cfblk3/1
  cfblk3/1 -> emi_789/1

== system sampleModel7293_pp_1_1/cfblk203/cfblk12/cfblk4 ==
  emi_1195 : Inport
  Action Port : ActionPort  ActionType=then
  cfblk4 : DiscreteFilter
  emi_1196 : Outport
  wires:
  emi_1195/1 -> cfblk4/1
  cfblk4/1 -> emi_1196/1

== system sampleModel7293_pp_1_1/cfblk203/cfblk12/cfblk5 ==
  emi_301 : Inport
  Action Port : ActionPort  ActionType=then
  cfblk5 : DiscreteStateSpace  SampleTime=-1
  emi_302 : Outport
  wires:
  emi_301/1 -> cfblk5/1
  cfblk5/1 -> emi_302/1

== system sampleModel7293_pp_1_1/cfblk203/cfblk12/cfblk9 ==
  emi_1571 : Inport
  emi_1572 : Inport  Port=2
  Action Port : ActionPort  ActionType=then
  cfblk9 : Delay  DelayLengthSource=Input port
      settings: InputPortMap=u0,p1
  emi_1573 : Outport
  wires:
  emi_1571/1 -> cfblk9/1
  emi_1572/1 -> cfblk9/2
  cfblk9/1 -> emi_1573/1

== system sampleModel7293_pp_1_1/cfblk203/cfblk12/emi_1197 ==
  Action Port : ActionPort  ActionType=else
  emi_1198 : Assertion

== system sampleModel7293_pp_1_1/cfblk203/cfblk12/emi_1268 ==
  Action Port : ActionPort  ActionType=else
  emi_1269 : Assertion

== system sampleModel7293_pp_1_1/cfblk203/cfblk12/emi_1574 ==
  Action Port : ActionPort  ActionType=else
  emi_1575 : Assertion

== system sampleModel7293_pp_1_1/cfblk203/cfblk12/emi_303 ==
  Action Port : ActionPort  ActionType=else
  emi_304 : Assertion

== system sampleModel7293_pp_1_1/cfblk203/cfblk12/emi_790 ==
  Action Port : ActionPort  ActionType=else
  emi_791 : Assertion

== system sampleModel7293_pp_1_1/cfblk203/cfblk13/cfblk11 ==
  emi_215 : Inport
  Action Port : ActionPort  ActionType=then
  cfblk11 : DiscreteFilter
  emi_216 : Outport
  wires:
  emi_215/1 -> cfblk11/1
  cfblk11/1 -> emi_216/1

== system sampleModel7293_pp_1_1/cfblk203/cfblk13/cfblk3 ==
  emi_129 : Inport
  Action Port : ActionPort  ActionType=then
  cfblk3 : Delay
  emi_130 : Outport
  wires:
  emi_129/1 -> cfblk3/1
  cfblk3/1 -> emi_130/1

== system sampleModel7293_pp_1_1/cfblk203/cfblk13/cfblk4 ==
  emi_1948 : Inport
  Action Port : ActionPort  ActionType=then
  cfblk4 : DiscreteStateSpace  SampleTime=-1
  emi_1949 : Outport
  wires:
  emi_1948/1 -> cfblk4/1
  cfblk4/1 -> emi_1949/1

== system sampleModel7293_pp_1_1/cfblk203/cfblk13/emi_131 ==
  Action Port : ActionPort  ActionType=else
  emi_132 : Assertion

== system sampleModel7293_pp_1_1/cfblk203/cfblk13/emi_1950 ==
  Action Port : ActionPort  ActionType=else
  emi_1951 : Assertion

== system sampleModel7293_pp_1_1/cfblk203/cfblk13/emi_217 ==
  Action Port : ActionPort  ActionType=else
  emi_218 : Assertion

== system sampleModel7293_pp_1_1/cfblk206/cfblk16/cfblk3 ==
  emi_1622 : Inport
  Action Port : ActionPort  ActionType=then
  cfblk3 : simulink/Discrete/Transfer Fcn Real Zero  ZeroZ=0.75  ICPrevInput=0.0  DoSatur=off
      settings: SourceProductName=Simulink  SourceProductBaseCode=SL
  emi_1623 : Outport
  wires:
  emi_1622/1 -> cfblk3/1
  cfblk3/1 -> emi_1623/1

== system sampleModel7293_pp_1_1/cfblk206/cfblk16/cfblk6 ==
  emi_1793 : Inport
  Action Port : ActionPort  ActionType=then
  cfblk6 : simulink/Discrete/Transfer Fcn Real Zero  ZeroZ=0.75  ICPrevInput=0.0  DoSatur=off
      settings: SourceProductName=Simulink  SourceProductBaseCode=SL
  emi_1794 : Outport
  wires:
  emi_1793/1 -> cfblk6/1
  cfblk6/1 -> emi_1794/1

== system sampleModel7293_pp_1_1/cfblk206/cfblk16/cfblk8 ==
  emi_2112 : Inport
  Action Port : ActionPort  ActionType=then
  cfblk8 : UnitDelay  SampleTime=-1
  emi_2113 : Outport
  wires:
  emi_2112/1 -> cfblk8/1
  cfblk8/1 -> emi_2113/1

== system sampleModel7293_pp_1_1/cfblk206/cfblk16/emi_1624 ==
  Action Port : ActionPort  ActionType=else
  emi_1625 : Assertion

== system sampleModel7293_pp_1_1/cfblk206/cfblk16/emi_1795 ==
  Action Port : ActionPort  ActionType=else
  emi_1796 : Assertion

== system sampleModel7293_pp_1_1/cfblk206/cfblk16/emi_2114 ==
  Action Port : ActionPort  ActionType=else
  emi_2115 : Assertion

== system sampleModel7293_pp_1_1/cfblk206/cfblk17/cfblk4 ==
  emi_1436 : Inport
  Action Port : ActionPort  ActionType=then
  cfblk4 : simulink/Discrete/Transfer Fcn Real Zero  ZeroZ=0.75  ICPrevInput=0.0  DoSatur=off
      settings: SourceProductName=Simulink  SourceProductBaseCode=SL
  emi_1437 : Outport
  wires:
  emi_1436/1 -> cfblk4/1
  cfblk4/1 -> emi_1437/1

== system sampleModel7293_pp_1_1/cfblk206/cfblk17/emi_1438 ==
  Action Port : ActionPort  ActionType=else
  emi_1439 : Assertion

== system sampleModel7293_pp_1_1/cfblk209/cfblk10/cfblk11 ==
  emi_1 : Inport
  Action Port : ActionPort  ActionType=then
  cfblk11 : simulink/Discrete/Transfer Fcn Lead or Lag  PoleZ=0.95  ZeroZ=0.75  ICPrevOutput=0.0  ICPrevInput=0.0  DoSatur=off
      settings: SourceProductName=Simulink  SourceProductBaseCode=SL
  emi_2 : Outport
  wires:
  emi_1/1 -> cfblk11/1
  cfblk11/1 -> emi_2/1

== system sampleModel7293_pp_1_1/cfblk209/cfblk10/emi_3 ==
  Action Port : ActionPort  ActionType=else
  emi_4 : Assertion

== system sampleModel7293_pp_1_1/cfblk209/cfblk9/cfblk11 ==
  emi_1899 : Inport
  Action Port : ActionPort  ActionType=then
  cfblk11 : UnitDelay  SampleTime=-1
  emi_1900 : Outport
  wires:
  emi_1899/1 -> cfblk11/1
  cfblk11/1 -> emi_1900/1

== system sampleModel7293_pp_1_1/cfblk209/cfblk9/cfblk17 ==
  emi_122 : Inport
  Action Port : ActionPort  ActionType=then
  cfblk17 : Delay
  emi_123 : Outport
  wires:
  emi_122/1 -> cfblk17/1
  cfblk17/1 -> emi_123/1

== system sampleModel7293_pp_1_1/cfblk209/cfblk9/cfblk4 ==
  emi_1230 : Inport
  Action Port : ActionPort  ActionType=then
  cfblk4 : simulink/Discrete/Transfer Fcn First Order  PoleZ=0.95  ICPrevOutput=0.0  DoSatur=off
      settings: SourceProductName=Simulink
  emi_1231 : Outport
  wires:
  emi_1230/1 -> cfblk4/1
  cfblk4/1 -> emi_1231/1

== system sampleModel7293_pp_1_1/cfblk209/cfblk9/emi_1232 ==
  Action Port : ActionPort  ActionType=else
  emi_1233 : Assertion

== system sampleModel7293_pp_1_1/cfblk209/cfblk9/emi_124 ==
  Action Port : ActionPort  ActionType=else
  emi_125 : Assertion

== system sampleModel7293_pp_1_1/cfblk209/cfblk9/emi_1901 ==
  Action Port : ActionPort  ActionType=else
  emi_1902 : Assertion

== system sampleModel7293_pp_1_1/cfblk210/cfblk18/cfblk4 ==
  emi_1579 : Inport
  Action Port : ActionPort  ActionType=then
  cfblk4 : simulink/Continuous/PID Controller  Controller=PID  TimeDomain=Discrete-time  SampleTime=-1  IntegratorMethod=Forward Euler  FilterMethod=Forward Euler  Form=Parallel  UseFilter=on  ControllerParametersSource=internal  P=1  I=1  D=0  N=100  InitialConditionSource=internal  InitialConditionForIntegrator=0  InitialConditionForFilter=0  ExternalReset=none  LimitOutput=off  UpperSaturationLimit=inf  LowerSaturationLimit=-inf  LinearizeAsGain=off  AntiWindupMode=none  Kb=1  TrackingMode=off  Kt=1  PParamMin=[]  PParamMax=[]  IParamMin=[]  IParamMax=[]  DParamMin=[]  DParamMax=[]  NParamMin=[]  NParamMax=[]  KbParamMin=[]  KbParamMax=[]  KtParamMin=[]  KtParamMax=[]  POutMin=[]  POutMax=[]  IOutMin=[]  IOutMax=[]  DOutMin=[]  DOutMax=[]  NOutMin=[]  NOutMax=[]  KbOutMin=[]  KbOutMax=[]  KtOutMin=[]  KtOutMax=[]  IntegratorOutMin=[]  IntegratorOutMax=[]  FilterOutMin=[]  FilterOutMax=[]  SumOutMin=[]  SumOutMax=[]  SumI1OutMin=[]  SumI1OutMax=[]  SumI2OutMin=[]  SumI2OutMax=[]  SumI3OutMin=[]  SumI3OutMax=[]  SumDOutMin=[]  SumDOutMax=[]  SaturationOutMin=[]  SaturationOutMax=[]  IntegratorContinuousStateAttributes=''  IntegratorStateMustResolveToSignalObject=off  IntegratorRTWStateStorageClass=Auto  FilterContinuousStateAttributes=''  FilterStateMustResolveToSignalObject=off  FilterRTWStateStorageClass=Auto  DifferentiatorICPrevScaledInput=0  DifferentiatorOutMin=[]  DifferentiatorOutMax=[]  FilterDiffOutCoefMin=[]  FilterDiffOutCoefMax=[]  SumDenOutMin=[]  SumDenOutMax=[]  SumNumOutMin=[]  SumNumOutMax=[]  ReciprocalOutMin=[]  ReciprocalOutMax=[]  DivideOutMin=[]  DivideOutMax=[]  TunerSelectOption=Transfer Function Based (PID Tuner App)
  emi_1580 : Outport
  wires:
  emi_1579/1 -> cfblk4/1
  cfblk4/1 -> emi_1580/1

== system sampleModel7293_pp_1_1/cfblk210/cfblk18/cfblk9 ==
  emi_1686 : Inport
  Action Port : ActionPort  ActionType=then
  cfblk9 : simulink/Discrete/Transfer Fcn Lead or Lag  PoleZ=0.95  ZeroZ=0.75  ICPrevOutput=0.0  ICPrevInput=0.0  DoSatur=off
      settings: SourceProductName=Simulink  SourceProductBaseCode=SL
  emi_1687 : Outport
  wires:
  emi_1686/1 -> cfblk9/1
  cfblk9/1 -> emi_1687/1

== system sampleModel7293_pp_1_1/cfblk210/cfblk18/emi_1581 ==
  Action Port : ActionPort  ActionType=else
  emi_1582 : Assertion

== system sampleModel7293_pp_1_1/cfblk210/cfblk18/emi_1688 ==
  Action Port : ActionPort  ActionType=else
  emi_1689 : Assertion

== system sampleModel7293_pp_1_1/cfblk213/cfblk14/cfblk12 ==
  emi_552 : Inport
  emi_553 : Inport  Port=2
  Action Port : ActionPort  ActionType=then
  cfblk12 : Delay  DelayLengthSource=Input port
      settings: InputPortMap=u0,p1
  emi_554 : Outport
  wires:
  emi_552/1 -> cfblk12/1
  emi_553/1 -> cfblk12/2
  cfblk12/1 -> emi_554/1

== system sampleModel7293_pp_1_1/cfblk213/cfblk14/cfblk16 ==
  emi_795 : Inport
  Action Port : ActionPort  ActionType=then
  cfblk16 : Delay
  emi_796 : Outport
  wires:
  emi_795/1 -> cfblk16/1
  cfblk16/1 -> emi_796/1

== system sampleModel7293_pp_1_1/cfblk213/cfblk14/cfblk17 ==
  emi_1100 : Inport
  Action Port : ActionPort  ActionType=then
  cfblk17 : Delay
  emi_1101 : Outport
  wires:
  emi_1100/1 -> cfblk17/1
  cfblk17/1 -> emi_1101/1

== system sampleModel7293_pp_1_1/cfblk213/cfblk14/cfblk19 ==
  emi_29 : Inport
  Action Port : ActionPort  ActionType=then
  cfblk19 : DataTypeConversion  OutDataTypeStr=double
  emi_30 : Outport
  wires:
  emi_29/1 -> cfblk19/1
  cfblk19/1 -> emi_30/1

== system sampleModel7293_pp_1_1/cfblk213/cfblk14/cfblk6 ==
  emi_588 : Inport
  emi_589 : Inport  Port=2
  Action Port : ActionPort  ActionType=then
  cfblk6 : Delay  ShowEnablePort=on
      settings: InputPortMap=u0,e6
  emi_590 : Outport
  wires:
  emi_588/1 -> cfblk6/1
  emi_589/1 -> cfblk6/2
  cfblk6/1 -> emi_590/1

== system sampleModel7293_pp_1_1/cfblk213/cfblk14/emi_1102 ==
  Action Port : ActionPort  ActionType=else
  emi_1103 : Assertion

== system sampleModel7293_pp_1_1/cfblk213/cfblk14/emi_31 ==
  Action Port : ActionPort  ActionType=else
  emi_32 : Assertion

== system sampleModel7293_pp_1_1/cfblk213/cfblk14/emi_555 ==
  Action Port : ActionPort  ActionType=else
  emi_556 : Assertion

== system sampleModel7293_pp_1_1/cfblk213/cfblk14/emi_591 ==
  Action Port : ActionPort  ActionType=else
  emi_592 : Assertion

== system sampleModel7293_pp_1_1/cfblk213/cfblk14/emi_797 ==
  Action Port : ActionPort  ActionType=else
  emi_798 : Assertion
